simulink model "Mass_spring"  (R2016a)
settings: Solver=VariableStepAuto  StartTime=0.0  StopTime=1000  RelTol=1e-3
undefined symbols (not defined in the file): b, k, M
settings Model: Creator=mm395  LastModifiedBy=mm395

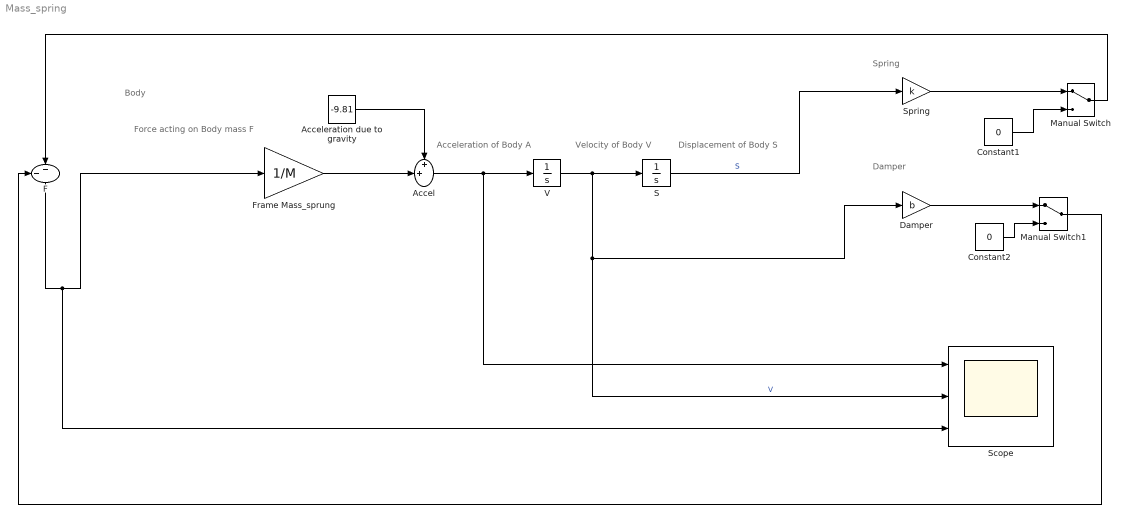
== system Mass_spring ==
  note: Body
  note: Acceleration of Body
      | A
  note: Force acting on Body mass
      | F
  note: Velocity of Body
      | V
  note: Displacement of Body
      | S
  note: Damper
  note: Spring
  Accel : Sum  Inputs=++|
  Acceleration due to gravity : Constant  Value=-9.81
  Constant1 : Constant  Value=0
  Constant2 : Constant  Value=0
  Damper : Gain  Gain=b
  F : Sum  Inputs=--|
  Frame Mass_sprung : Gain  Gain=1/M
  Manual Switch : ManualSwitch
  Manual Switch1 : ManualSwitch
  S : Integrator
  Scope : Scope  NumInputPorts=3
  Spring : Gain  Gain=k
  V : Integrator
  wires:
  Frame Mass_sprung/1 -> Accel/2
  Acceleration due to gravity/1 -> Accel/1
  V/1 -> Damper/1, Scope/2, S/1  "V"
  Accel/1 -> Scope/1, V/1
  S/1 -> Spring/1  "S"
  F/1 -> Frame Mass_sprung/1, Scope/3
  Spring/1 -> Manual Switch/1
  Damper/1 -> Manual Switch1/1
  Manual Switch/1 -> F/2
  Manual Switch1/1 -> F/1
  Constant1/1 -> Manual Switch/2
  Constant2/1 -> Manual Switch1/2
